simulink model "Engine_10V"  (R2023a)
settings: Solver=VariableStepAuto  StartTime=0.0  StopTime=10.0  RelTol=1e-3
values from neighbouring files (symbols this model uses):
  Cm = 1.3    [Init.m]
  Cw = 3.15    [Init.m]
  J = 0.000007    (= 7e-06)    [Init.m]
  Lob = 0.013    [Init.m]
  Lya = 0.0015    [Init.m]
  Rya = 8    [Init.m]
settings Model: Creator=Waffle  LastModifiedBy=Waffle

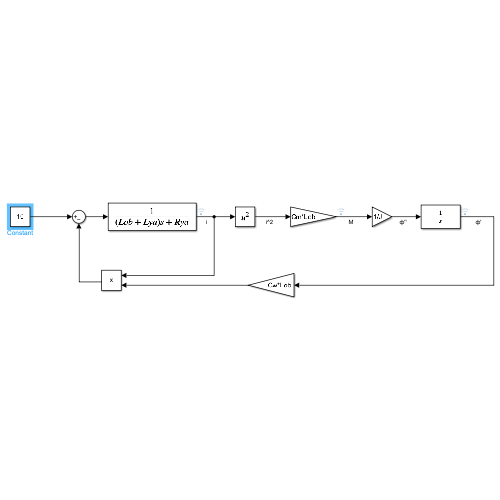
[thumbnail: Simulink's stored preview of the top-level diagram]
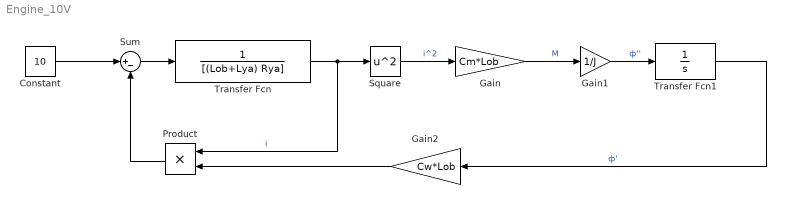
== system Engine_10V ==
  Constant : Constant  Value=10
  Gain : Gain  Gain=Cm*Lob
  Gain1 : Gain  Gain=1/J
  Gain2 : Gain  Gain=Cw*Lob
  Product : Product
  Square : Math  Operator=square
  Sum : Sum  Inputs=|+-
  Transfer Fcn : TransferFcn  Denominator=[(Lob+Lya) Rya]
  Transfer Fcn1 : TransferFcn  Denominator=[1 0]
  wires:
  Constant/1 -> Sum/1
  Sum/1 -> Transfer Fcn/1
  Transfer Fcn/1 -> Product/1, Square/1  "i"
  Square/1 -> Gain/1  "i^2"
  Gain/1 -> Gain1/1  "М"
  Gain1/1 -> Transfer Fcn1/1  "ф''"
  Product/1 -> Sum/2
  Transfer Fcn1/1 -> Gain2/1  "ф'"
  Gain2/1 -> Product/2
